simulink library "Lib_DQTrans_dqs2dqeProductT"  (R2021a)
settings: Solver=VariableStepAuto  StartTime=0.0  StopTime=10.0  RelTol=1e-3
settings Model: Creator=30610  LastModifiedBy=30610

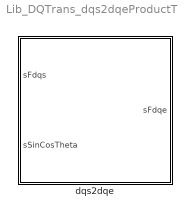
== system Lib_DQTrans_dqs2dqeProductT ==
  dqs2dqe : Subsystem

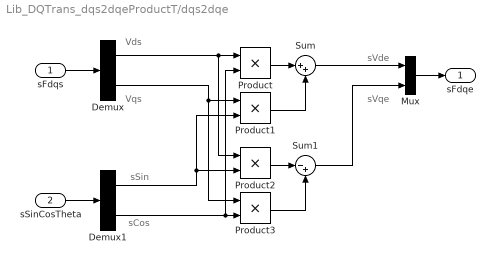
== system Lib_DQTrans_dqs2dqeProductT/dqs2dqe ==
  note: sVqe
  note: sVde
  note: sCos
  note: sSin
  note: Vqs
  note: Vds
  sFdqs : Inport
  sSinCosTheta : Inport  Port=2
  Demux : Demux  Outputs=2
  Demux1 : Demux  Outputs=2
  Mux : Mux  Inputs=2
  Product{,1..3} (4 alike) : Product  RndMeth=Zero
  Sum : Sum  Inputs=|++
  Sum1 : Sum  Inputs=|-+
  sFdqe : Outport  VectorParamsAs1DForOutWhenUnconnected=off
  wires:
  Product/1 -> Sum/1
  Product3/1 -> Sum1/2
  Demux/1 -> Product2/1, Product/1
  Demux1/2 -> Product/2, Product3/2
  sFdqs/1 -> Demux/1
  Demux1/1 -> Product1/2, Product2/2
  Product1/1 -> Sum/2
  Demux/2 -> Product3/1, Product1/1
  Product2/1 -> Sum1/1
  Mux/1 -> sFdqe/1
  sSinCosTheta/1 -> Demux1/1
  Sum/1 -> Mux/1
  Sum1/1 -> Mux/2
